simulink library "slstlib"  (R2015a)
settings: Solver=ode45  StartTime=0.0  StopTime=10.0  RelTol=1e-3
undefined symbols (not defined in the file): phi
libraries: simulink x5
settings Model: Creator=alex  LastModifiedBy=donze

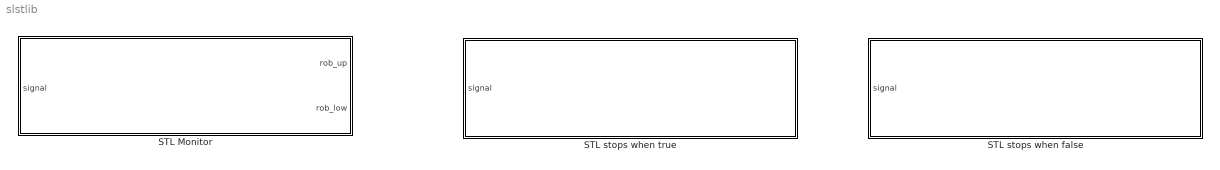
== system slstlib ==
  STL Monitor : Subsystem  mask{SignalNames='x1,x2', STLString='x1[t]>0', MaxRob=100, RefreshRate=0.1, rob_low_lim=inf, rob_up_lim=-inf, rob_diff_lim=-inf}
      mask prompts: SignalNames "Signal names"; STLString "Enter STL formula (string)"; MaxRob "Enter max abs value of signals"; RefreshRate "Monitoring refresh rate"; rob_low_lim "Stops when satisfaction is above"; rob_up_lim "Stops when satisfaction is below"; rob_diff_lim "Stops when satisfaction interval is less than"
      mask Display:
      | st_len = numel(STLString);
      | fprintf('Interval satisfaction at time 0 of:\n%s     ', STLString(1:min(st_len, 40)))
      | 
      | % label output ports
      | port_label('output',1,'\rho_{up}', 'Interpreter', 'tex')
      | port_label('output',2,'\rho_{low}', 'Interpreter', 'tex')
      | 
      | % label input ports
      | split = strsplit(SignalNames,',');
      | nbdim = numel(split);
      | in_label = sprintf('%d-dim:',nbdim);
      | for il= 1:nbdim
      |    in_label = sprintf([in_label '\n' split{il}]);
      | end
      | 
      | port_label('input',1, in_label);
  STL stops when false : Subsystem  mask{SignalNames='x1,x2', STLString='x1[t]>0', MaxRob=100, Tstart=0, Tend=100, RefreshRate=0.1, rob_up_lim=0}
      mask prompts: SignalNames "Signal names"; STLString "STL formula"; MaxRob "Max abs value of signals"; Tstart "Start time"; Tend "End time"; RefreshRate "Monitoring refresh rate"; rob_up_lim "Stops when satisfaction is below"
      mask Display:
      | st_len = numel(STLString);
      | fprintf('Stops simulation when true in [%g,%g]:\n%s', Tstart, Tend, STLString(1:min(st_len, 40)))
      | 
      | % label input ports
      | split = strsplit(SignalNames,',');
      | nbdim = numel(split);
      | in_label = sprintf('%d-dim:',nbdim);
      | for il= 1:nbdim
      |    in_label = sprintf([in_label '\n' split{il}]);
      | end
      | 
      | port_label('input',1, in_label);
  STL stops when true : Subsystem  mask{SignalNames='x1,x2', STLString='x1[t]>0', MaxRob=100, Tstart=0, Tend=100, RefreshRate=0.1, rob_low_lim=0}
      mask prompts: SignalNames "Signal names"; STLString "STL formula"; MaxRob "Max abs value of signals"; Tstart "Start time"; Tend "End time"; RefreshRate "Monitoring refresh rate"; rob_low_lim "Stops when satisfaction is above"
      mask Display:
      | st_len = numel(STLString);
      | fprintf('Stops simulation when true in [%g,%g]:\n%s', Tstart, Tend, STLString(1:min(st_len, 40)))
      | 
      | % label input ports
      | split = strsplit(SignalNames,',');
      | nbdim = numel(split);
      | in_label = sprintf('%d-dim:',nbdim);
      | for il= 1:nbdim
      |    in_label = sprintf([in_label '\n' split{il}]);
      | end
      | 
      | port_label('input',1, in_label);

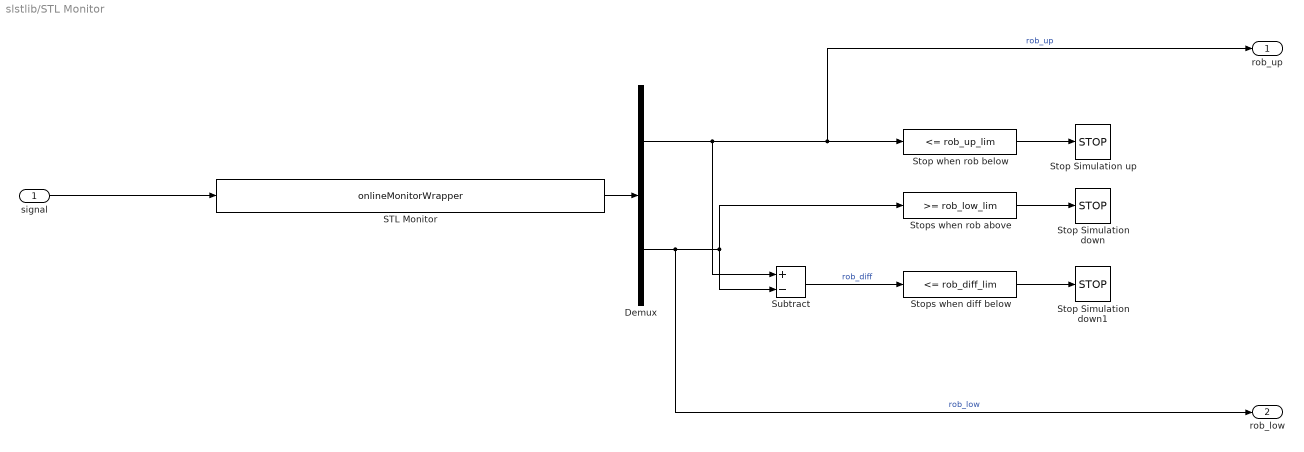
== system slstlib/STL Monitor ==
  signal : Inport
  Demux : Demux  Outputs=2
  "STL Monitor " : S-Function  FunctionName=onlineMonitorWrapper  Parameters=SignalNames, STLString, MaxRob, RefreshRate  mask(STL Monitor){SignalNames=SignalNames, STLString=phi, MaxRob=MaxRob, RefreshRate=RefreshRate}
      mask prompts: SignalNames "Signal names"; STLString "String For STL formula"; MaxRob "Maximum robustness"; RefreshRate "Refresh Rate"
      mask help:
      | Monitor an STL Formula on input signal. Takes two parameters: a string with
      | comma separated identifiers for the input signals, (ex: 'x1,x2,y'), and a
      | string for the formula (ex: 'alw_[0, 50] (x1[t]>0 => y[t] >0)'). Outputs a
      | two dimensional signal bounding the satisfaction of the formula.
      mask Display: fprintf('%s', STLString)
  Stop Simulation down : Stop
  Stop Simulation down1 : Stop
  Stop Simulation up : Stop
  Stop when rob below : simulink/Logic and Bit Operations/Compare To Constant  relop=<=  const=rob_up_lim  OutDataTypeStr=boolean
  Stops when diff below : simulink/Logic and Bit Operations/Compare To Constant  relop=<=  const=rob_diff_lim  OutDataTypeStr=boolean
  Stops when rob above : simulink/Logic and Bit Operations/Compare To Constant  relop=>=  const=rob_low_lim  OutDataTypeStr=boolean
  Subtract : Sum  Inputs=+-
  rob_up : Outport
  rob_low : Outport  Port=2
  wires:
  Demux/2 -> rob_low/1, Stops when rob above/1, Subtract/2  "rob_low"
  "STL Monitor "/1 -> Demux/1
  Stops when rob above/1 -> Stop Simulation down/1
  Demux/1 -> Subtract/1, rob_up/1, Stop when rob below/1  "rob_up"
  Subtract/1 -> Stops when diff below/1  "rob_diff"
  Stops when diff below/1 -> Stop Simulation down1/1
  signal/1 -> "STL Monitor "/1
  Stop when rob below/1 -> Stop Simulation up/1

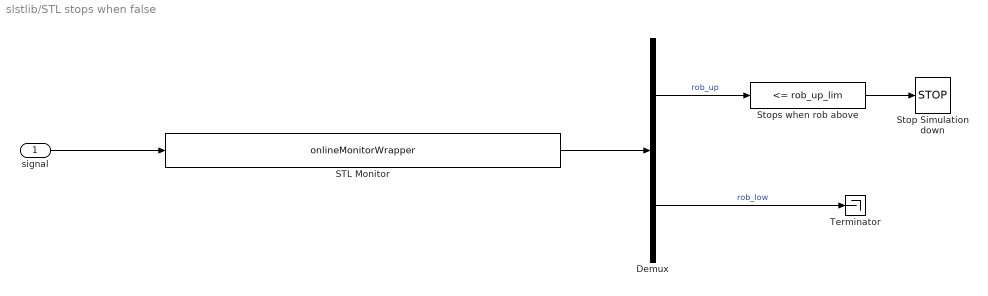
== system slstlib/STL stops when false ==
  signal : Inport
  Demux : Demux  Outputs=2
  "STL Monitor " : S-Function  FunctionName=onlineMonitorWrapper  Parameters=SignalNames, STLString, MaxRob, RefreshRate  mask(STL Monitor){SignalNames=SignalNames, STLString=['alw_[' num2str(Tstart) ', ' num2str(Tend) '] ' STLString], MaxRob=MaxRob, RefreshRate=RefreshRate}
      mask prompts: SignalNames "Signal names"; STLString "String For STL formula"; MaxRob "Maximum robustness"; RefreshRate "Refresh Rate"
      mask help:
      | Monitor an STL Formula on input signal. Takes two parameters: a string with
      | comma separated identifiers for the input signals, (ex: 'x1,x2,y'), and a
      | string for the formula (ex: 'alw_[0, 50] (x1[t]>0 => y[t] >0)'). Outputs a
      | two dimensional signal bounding the satisfaction of the formula.
      mask Display: fprintf('%s', STLString)
  Stop Simulation down : Stop
  Stops when rob above : simulink/Logic and Bit Operations/Compare To Constant  relop=<=  const=rob_up_lim  OutDataTypeStr=boolean
  Terminator : Terminator
  wires:
  Demux/1 -> Stops when rob above/1  "rob_up"
  Demux/2 -> Terminator/1  "rob_low"
  "STL Monitor "/1 -> Demux/1
  Stops when rob above/1 -> Stop Simulation down/1
  signal/1 -> "STL Monitor "/1

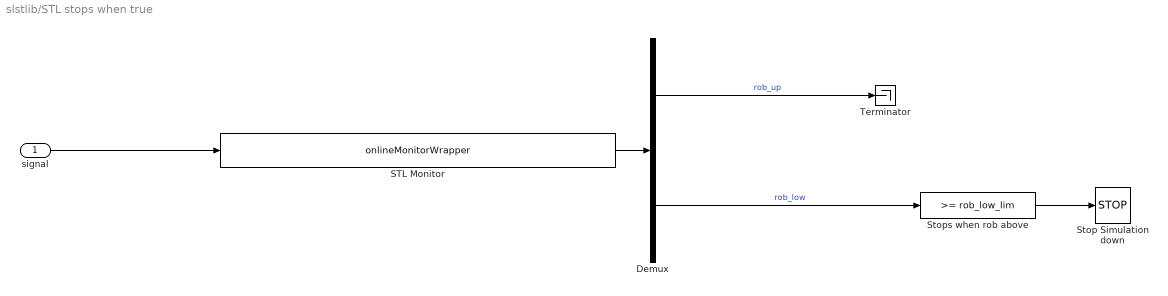
== system slstlib/STL stops when true ==
  signal : Inport
  Demux : Demux  Outputs=2
  "STL Monitor " : S-Function  FunctionName=onlineMonitorWrapper  Parameters=SignalNames, STLString, MaxRob, RefreshRate  mask(STL Monitor){SignalNames=SignalNames, STLString=['ev_[' num2str(Tstart) ', ' num2str(Tend) '] ' STLString], MaxRob=MaxRob, RefreshRate=RefreshRate}
      mask prompts: SignalNames "Signal names"; STLString "String For STL formula"; MaxRob "Maximum robustness"; RefreshRate "Refresh Rate"
      mask help:
      | Monitor an STL Formula on input signal. Takes two parameters: a string with
      | comma separated identifiers for the input signals, (ex: 'x1,x2,y'), and a
      | string for the formula (ex: 'alw_[0, 50] (x1[t]>0 => y[t] >0)'). Outputs a
      | two dimensional signal bounding the satisfaction of the formula.
      mask Display: fprintf('%s', STLString)
  Stop Simulation down : Stop
  Stops when rob above : simulink/Logic and Bit Operations/Compare To Constant  relop=>=  const=rob_low_lim  OutDataTypeStr=boolean
  Terminator : Terminator
  wires:
  signal/1 -> "STL Monitor "/1
  Stops when rob above/1 -> Stop Simulation down/1
  "STL Monitor "/1 -> Demux/1
  Demux/2 -> Stops when rob above/1  "rob_low"
  Demux/1 -> Terminator/1  "rob_up"
